simulink model "phase2_scheduler_testbed"  (R2026a)
settings: Solver=VariableStepAuto  StopTime=0.15  FixedStep=0.01  EnableMultiTasking=on
undefined symbols (not defined in the file): D1, D2, D3, P
libraries: proctasklib x1
settings Model: Creator=The MathWorks, Inc.  LastModifiedBy=rayyu
settings SolverCC: PositivePriorityOrder=on
settings HardwareCC: ProdBitPerLong=64.0  ProdLargestAtomicInteger=LongLong  ProdLargestAtomicFloat=Double  ProdHWDeviceType=ARM Compatible->ARM Cortex-A (64-bit)  HardwareBoardFeatureSet=SoCBlockset
settings RTWCC: SystemTargetFile=ert.tlc  HardwareBoard=Xilinx Zynq UltraScale+ MPSoC ZCU102 Evaluation Kit  TLCOptions="-aInlineSetEventsForThisBaseRateFcn=TLC_FALSE -aSuppressMultiTaskScheduler=TLC_FALSE  -aRateBasedStepFcn=0"  GenerateReport=on  Toolchain=Linaro AArch64 Linux v6.3.1  IncludeHyperlinkInReport=on  LaunchReport=on  GenerateTraceInfo=on  GenerateTraceReport=on  GenerateTraceReportSl=on  GenerateTraceReportSf=on  GenerateTraceReportEml=on  Description=Embedded Coder
settings ERTTargetCC: ExtModeTransport=2.0  DynamicArrayContainerType=coder::array

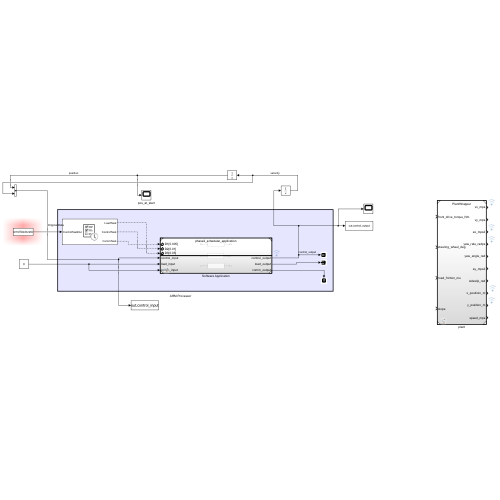
[thumbnail: Simulink's stored preview of the top-level diagram]
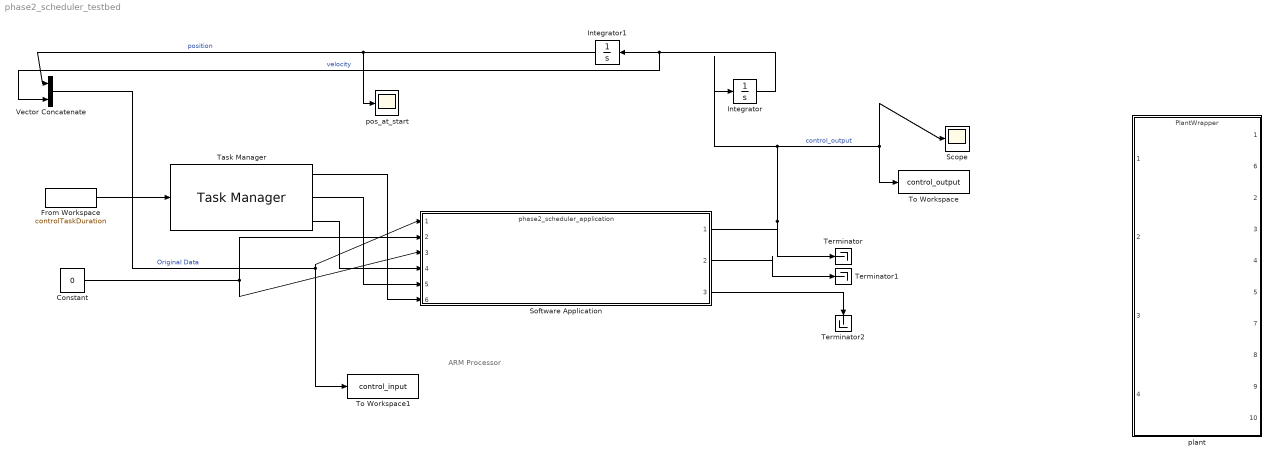
== system phase2_scheduler_testbed ==
  note: ARM Processor
  Constant : Constant  Value=0
  From Workspace : FromWorkspace  VariableName=controlTaskDuration  Interpolate=off  OutputAfterFinalValue=Holding final value
  Integrator : Integrator
  Integrator1 : Integrator  InitialCondition=1
  Scope : Scope
      settings: ActiveDisplayYMinimum=-2.25  ActiveDisplayYMaximum=0.24999999999999994
  Software Application : ModelReference  ModelNameDialog=phase2_scheduler_application.slx  SimulationMode=Normal  ScheduleRates=on  CachedPortDiscreteRates=[0.005;0.01;0.05]  ModelEventPortInfo=P:D1[0.005][0][0],P:D2[0.01][0][0],P:D3[0.05][0][0]  ModelReferenceVersion=14.11
  Task Manager : proctasklib/Task Manager  AllTaskData="[{\"taskName\":\"LoadTask\",\"taskType\":\"Timer-driven\",\"taskEvent\":\"LoadTaskEvent\",\"taskPeriod\":\"0.05\",\"taskPriority\":\"50\",\"coreSelection\":\"Specified core\",\"coreNum\":\"0\",\"dropOverranTasks\":false,\"playbackRecorded\":false,\"diagnosticsFile\":\"\",\"taskDurationSource\":\"Dialog\",\"taskDuration\":1E-6,\"taskDurationDeviation\":0,\"logExecutionData\":true,\"logDroppedTasks\":false,\"version\":\"2.6\",\"taskDurationData\":{\"percent\":\"100\",\"mean\":\"0.03\",\"dev\":\"0\",\"min\":\"0.03\",\"max\":\"0.03\"},\"taskEventSource\":\"Internal\",\"taskEventSourceAssignmentType\":\"AutoAssigned\",\"taskEventSourceType\":\"Unspecified\",\"taskEventGroup\":\"Unspecified\",\"taskEventInterrupt\":\"Unspecified\",\"taskEventOrder\":1,\"taskDisablePremption\":false,\"taskClearInterruptFlagsAtEndOfEvent\":false},{\"taskName\":\"ControlTask\",\"taskType\":\"Timer-driven\",\"taskEvent\":\"ControlTaskEvent\",\"taskPeriod\":\"0.01\",\"taskPriority\":\"50\",\"coreSelection\":\"Specified core\",\"coreNum\":\"0\",\"dropOverranTasks\":false,\"playbackRecorded\":false,\"diagnosticsFile\":\"\",\"taskDurationSource\":\"Input port\",\"taskDuration\":1E-6,\"taskDurationDeviation\":0,\"logExecutionData\":true,\"logDroppedTasks\":false,\"version\":\"2.6\",\"taskDurationData\":{\"percent\":\"100\",\"mean\":\"0.003\",\"dev\":\"0\",\"min\":\"0.003\",\"max\":\"0.003\"},\"taskEventSource\":\"Internal\",\"taskEventSourceAssignmentType\":\"AutoAssigned\",\"taskEventSourceType\":\"Unspecified\",\"taskEventGroup\":\"Unspecified\",\"taskEventInterrupt\":\"Unspecified\",\"taskEventOrder\":1,\"taskDisablePremption\":false,\"taskClearInterruptFlagsAtEndOfEvent\":false},{\"taskName\":\"CommTask\",\"taskType\":\"Timer-driven\",\"taskEvent\":\"CommTaskEvent\",\"taskPeriod\":\"0.005\",\"taskPriority\":\"50\",\"coreSelection\":\"Specified core\",\"coreNum\":\"0\",\"dropOverranTasks\":false,\"playbackRecorded\":false,\"diagnosticsFile\":\"\",\"taskDurationSource\":\"Dialog\",\"taskDuration\":1E-6,\"taskDurationDeviation\":0,\"logExecutionData\":true,\"logDroppedTasks\":false,\"version\":\"2.6\",\"taskDurationData\":{\"percent\":\"100\",\"mean\":\"0.0005\",\"dev\":\"0\",\"min\":\"0.0005\",\"max\":\"0.0005\"},\"taskEventSource\":\"Internal\",\"taskEventSourceAssignmentType\":\"AutoAssigned\",\"taskEventSourceType\":\"Unspecified\",\"taskEventGroup\":\"Unspecified\",\"taskEventInterrupt\":\"Unspecified\",\"taskEventOrder\":1,\"taskDisablePremption\":false,\"taskClearInterruptFlagsAtEndOfEvent\":false}]"  EnableTaskSimulation=on  StreamToSDI=on  WriteToFile=off  OverwriteFile=off  SupportEventPorts=on  UseScheduleEditor=off  CustomizationInfo=''
  Terminator : Terminator
  Terminator1 : Terminator
  Terminator2 : Terminator
  To Workspace : ToWorkspace  VariableName=control_output  SaveFormat=Timeseries  SampleTime=-1
  To Workspace1 : ToWorkspace  VariableName=control_input  SaveFormat=Timeseries  SampleTime=-1
  Vector Concatenate : Concatenate
  plant : ModelReference  ModelNameDialog=PlantWrapper.slx  SimulationMode=Normal  ModelReferenceVersion=1.23
      settings: PortSchema="{\"entries\":[{\"content\":{\"sides\":[{\"content\":{\"connectorIds\":[\"In1\",\"In2\",\"In3\",\"In4\"]},\"type\":\"ConnectorPlacement.EquallySpacedRectSide\",\"uuid\":\"bf665537-3fd8-4fa0-88a8-2cb308153754\"},{\"content\":{\"connectorIds\":[\"Out1\",\"Out6\",\"Out2\",\"Out3\",\"Out4\",\"Out5\",\"Out7\",\"Out8\",\"Out9\",\"Out10\"],\"side\":\"RIGHT\"},\"type\":\"ConnectorPlacement.EquallySpacedRectSide\",\"uuid\":\"a274990e-adc2-49b8-8679-a2f39e53ce6e\"},{\"content\":{\"side\":\"TOP\"},\"type\":\"ConnectorPlacement.EquallySpacedRectSide\",\"uuid\":\"963f9bff-e020-46b1-9958-cad0758083aa\"}]},\"type\":\"ConnectorPlacement.EquallySpacedConnector\",\"uuid\":\"fb8d0fca-1617-49ee-84dd-83e8b757a297\"}],\"packageUris\":[\"http://schema.mathworks.com/mf0/Connector/R2020b\"],\"version\":\"1.0\"}"
  pos_at_start : Scope
      settings: ActiveDisplayYMinimum=0.9805911383257554  ActiveDisplayYMaximum=1.0067345814965289
  wires:
  Software Application/1 -> Terminator/1, Scope/1, To Workspace/1, Integrator/1  "control_output"
  Vector Concatenate/1 -> To Workspace1/1, Software Application/1  "Original Data"
  Task Manager/1 -> Software Application/6
  Software Application/2 -> Terminator1/1
  Constant/1 -> Software Application/3, Software Application/2
  Integrator/1 -> Vector Concatenate/2, Integrator1/1  "velocity"
  Integrator1/1 -> pos_at_start/1, Vector Concatenate/1  "position"
  Task Manager/2 -> Software Application/5
  Software Application/3 -> Terminator2/1
  Task Manager/3 -> Software Application/4
  From Workspace/1 -> Task Manager/1
